simulink model "SimpleNonStablePlant"  (R2023b)
settings: Solver=VariableStepAuto  StartTime=0.0  StopTime=100  RelTol=1e-3
libraries: dspsrcs4 x2
settings Model: Creator=Alex  LastModifiedBy=Alex

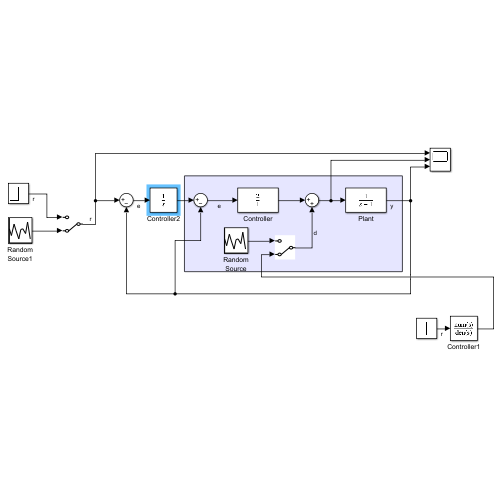
[thumbnail: Simulink's stored preview of the top-level diagram]
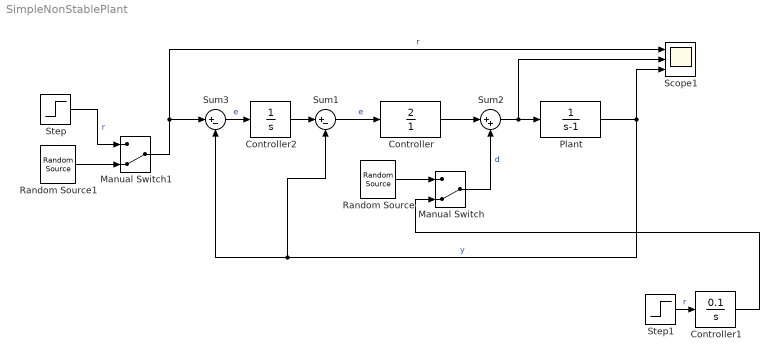
== system SimpleNonStablePlant ==
  Controller : TransferFcn  Numerator=[2]  Denominator=[1]
  Controller1 : TransferFcn  Numerator=[0.1]  Denominator=[1 0]
  Controller2 : TransferFcn  Denominator=[1 0]
  Manual Switch : ManualSwitch  CurrentSetting=0
  Manual Switch1 : ManualSwitch  CurrentSetting=0
  Plant : TransferFcn  Denominator=[1 -1]
  Random Source : dspsrcs4/Random Source  SrcType=Uniform  NormMethod=Ziggurat  CltLength=12  MinVal=-0.1  MaxVal=0.1  MeanVal=0  VarVal=1  RepMode=Not repeatable  rawSeed=1  IsInherit=off  SampMode=Discrete  SampTime=0.1  SampFrame=1  DataType=Double  OutComplex=Real  OutputFrames=off
  Random Source1 : dspsrcs4/Random Source  SrcType=Uniform  NormMethod=Ziggurat  CltLength=12  MinVal=-1  MaxVal=1  MeanVal=0  VarVal=1  RepMode=Not repeatable  rawSeed=1  IsInherit=off  SampMode=Discrete  SampTime=10  SampFrame=1  DataType=Double  OutComplex=Real  OutputFrames=off
  Scope1 : Scope  NumInputPorts=3
  Step : Step  SampleTime=0
  Step1 : Step  SampleTime=0
  Sum1 : Sum  Inputs=|+-
  Sum2 : Sum  Inputs=|++
  Sum3 : Sum  Inputs=|+-
  wires:
  Controller/1 -> Sum2/1
  Sum1/1 -> Controller/1  "e"
  Plant/1 -> Sum1/2, Sum3/2, Scope1/3  "y"
  Random Source/1 -> Manual Switch/1
  Sum2/1 -> Scope1/2, Plant/1
  Manual Switch/1 -> Sum2/2  "d"
  Controller2/1 -> Sum1/1
  Manual Switch1/1 -> Scope1/1, Sum3/1  "r"
  Random Source1/1 -> Manual Switch1/2
  Step/1 -> Manual Switch1/1  "r"
  Sum3/1 -> Controller2/1  "e"
  Step1/1 -> Controller1/1  "r"
  Controller1/1 -> Manual Switch/2
